simulink model "SensorFusion_Controller_Model"  (R2025a)
settings: Solver=VariableStepAuto  StartTime=0.0  StopTime=inf  FixedStep=1  RelTol=1e-3
undefined symbols (not defined in the file): DiscIntNeverNeededParam
libraries: simulink x17
(part 2 of 4)

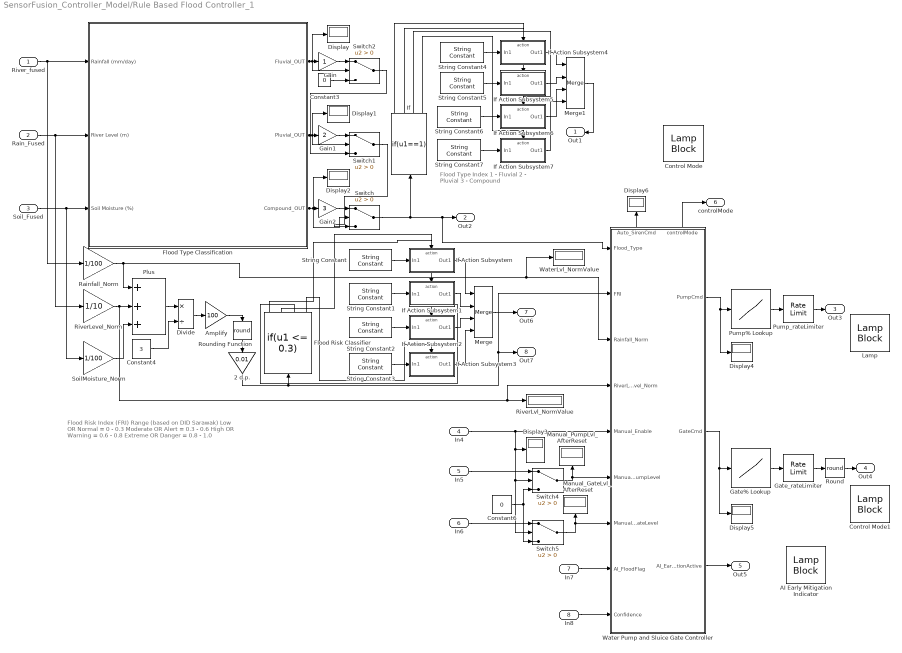
== system SensorFusion_Controller_Model/Rule Based Flood Controller_1 ==
  note: Flood Risk Index (FRI) Range (based on DID Sarawak)
      |
      | Low OR		Normal = 0 - 0.3
      | Moderate OR	Alert = 0.3 - 0.6
      | High OR		Warning = 0.6 - 0.8
      | Extreme OR 	Danger = 0.8 - 1.0
  note: Flood Type Index
      | 1 - Fluvial
      | 2 - Pluvial
      | 3 - Compound
  River_fused : Inport
  Rain_Fused : Inport  Port=2
  Soil_Fused : Inport  Port=3
  In4 : Inport  Port=4
  In5 : Inport  Port=5
  In6 : Inport  Port=6
  In7 : Inport  Port=7
  In8 : Inport  Port=8
  2 d.p. : Gain  Gain=0.01
  AI Early Mitigation Indicator : LampBlock  LabelPosition=Hide  DefaultColor=[192.0, 192.0, 192.0]
  Amplify : Gain  Gain=100
  Constant3 : Constant  Value=0
  Constant4 : Constant  Value=3
  Constant6 : Constant  Value=0
  Control Mode : LampBlock  LabelPosition=Hide  DefaultColor=[192.0, 192.0, 192.0]
  Control Mode1 : LampBlock  LabelPosition=Hide  DefaultColor=[192.0, 192.0, 192.0]
  Display{,1..6} (7 alike) : Display
  Divide : Product  Inputs=*/
  Flood Risk Classifier : If  IfExpression=u1 <= 0.3  ElseIfExpressions=u1 <= 0.6,u1 < 0.8
  Flood Type Classification : Subsystem
  Gain : Gain
  Gain1 : Gain  Gain=2
  Gain2 : Gain  Gain=3
  Gate% Lookup : Lookup_n-D  NumberOfTableDimensions=1  BreakpointsForDimension1=[0 1 2 3]  Table=[0 30 70 100]  InternalRulePriority=Speed  RndMeth=Simplest
  Gate_rateLimiter : RateLimiter  SampleTimeMode=inherited
  If : If  IfExpression=u1==1  ElseIfExpressions=u1==2,u1==3
  If Action Subsystem : Subsystem  TreatAsAtomicUnit=on
  If Action Subsystem1 : Subsystem  TreatAsAtomicUnit=on
  If Action Subsystem2 : Subsystem  TreatAsAtomicUnit=on
  If Action Subsystem3 : Subsystem  TreatAsAtomicUnit=on
  If Action Subsystem4 : Subsystem  TreatAsAtomicUnit=on
  If Action Subsystem5 : Subsystem  TreatAsAtomicUnit=on
  If Action Subsystem6 : Subsystem  TreatAsAtomicUnit=on
  If Action Subsystem7 : Subsystem  TreatAsAtomicUnit=on
  Lamp : LampBlock  LabelPosition=Hide  DefaultColor=[192.0, 192.0, 192.0]
  Manual_GateLvl_AfterReset : Display
  Manual_PumpLvl_AfterReset : Display
  Merge : Merge  Inputs=4
  Merge1 : Merge  Inputs=4
  Plus : Sum  Inputs=+++
  Pump% Lookup : Lookup_n-D  NumberOfTableDimensions=1  BreakpointsForDimension1=[0 1 2 3]  Table=[0 30 70 100]  InternalRulePriority=Speed  RndMeth=Simplest
  Pump_rateLimiter : RateLimiter  RisingSlewLimit=20  FallingSlewLimit=-30  SampleTimeMode=inherited
  Rainfall_Norm : Gain  Gain=1/100
  RiverLevel_Norm : Gain  Gain=1/10
  RiverLvl_NormValue : Display
  Round : Rounding  Operator=round
  Rounding Function : Rounding  Operator=round
  SoilMoisture_Norm : Gain  Gain=1/100
  String Constant : StringConstant  String="\"NORMAL\""
  String Constant1 : StringConstant  String="\"ALERT\""
  String Constant2 : StringConstant  String="\"WARNING\""
  String Constant3 : StringConstant  String="\"DANGER\""
  String Constant4 : StringConstant  String="\"FLUVIAL\""
  String Constant5 : StringConstant  String="\"PLUVIAL\""
  String Constant6 : StringConstant  String="\"COMPOUND\""
  String Constant7 : StringConstant  String="\"SAFE\""
  Switch{,1..2,4..5} (5 alike) : Switch  Criteria=u2 > Threshold  SaturateOnIntegerOverflow=off  InputSameDT=off
  Water Pump and Sluice Gate Controller : Stateflow chart  TreatAsAtomicUnit=on
      settings: PortSchema="{\"entries\":[{\"content\":{\"sides\":[{\"content\":{\"connectorIds\":[\"In2\",\"In1\",\"In8\",\"In9\",\"In3\",\"In5\",\"In4\",\"In6\",\"In7\"]},\"type\":\"ConnectorPlacement.EquallySpacedRectSide\",\"uuid\":\"f2c8d520-50f7-4f0f-a2cf-48793db073c2\"},{\"content\":{\"connectorIds\":[\"Out1\",\"Out2\",\"Out5\"],\"side\":\"RIGHT\"},\"type\":\"ConnectorPlacement.EquallySpacedRectSide\",\"uuid\":\"5649f6ce-feb7-45bc-b5a3-9e67182959d5\"},{\"content\":{\"connectorIds\":[\"Out3\",\"Out4\"],\"side\":\"TOP\"},\"type\":\"ConnectorPlacement.EquallySpacedRectSide\",\"uuid\":\"5d953d1b-f348-4b99-981e-4266d38d1676\"}]},\"type\":\"ConnectorPlacement.EquallySpacedConnector\",\"uuid\":\"2b0f672a-dc23-486c-8ba1-c7509a856d5e\"}],\"packageUris\":[\"http://schema.mathworks.com/mf0/Connector/R2020b\"],\"version\":\"1.0\"}"
  WaterLvl_NormValue : Display
  Out1 : Outport
  Out2 : Outport  Port=2
  Out3 : Outport  Port=3
  Out4 : Outport  Port=4
  Out5 : Outport  Port=5
  controlMode : Outport  Port=6
  Out6 : Outport  Port=7
  Out7 : Outport  Port=8
  wires:
  If/3 -> If Action Subsystem6/Action
  RiverLevel_Norm/1 -> Plus/2, RiverLvl_NormValue/1, Water Pump and Sluice Gate Controller/9(RiverLevel_Norm)
  String Constant2/1 -> If Action Subsystem2/1(In1)
  Flood Risk Classifier/2 -> If Action Subsystem1/Action
  If Action Subsystem3/1(Out1) -> Merge/4
  Soil_Fused/1 -> SoilMoisture_Norm/1, Flood Type Classification/3(Soil Moisture (%))
  Rain_Fused/1 -> RiverLevel_Norm/1, Flood Type Classification/2(River Level (m))
  String Constant1/1 -> If Action Subsystem1/1(In1)
  Flood Risk Classifier/4 -> If Action Subsystem3/Action
  If Action Subsystem7/1(Out1) -> Merge1/4
  In7/1 -> Water Pump and Sluice Gate Controller/6(AI_FloodFlag)
  Amplify/1 -> Rounding Function/1
  Constant3/1 -> Switch2/3
  Merge1/1 -> Out1/1
  Water Pump and Sluice Gate Controller/1(PumpCmd) -> Display4/1, Pump% Lookup/1
  Water Pump and Sluice Gate Controller/5(AI_EarlyMitigationActive) -> Out5/1
  Switch4/1 -> Water Pump and Sluice Gate Controller/5(Manual_PumpLevel), Manual_PumpLvl_AfterReset/1
  String Constant5/1 -> If Action Subsystem5/1(In1)
  String Constant3/1 -> If Action Subsystem3/1(In1)
  Flood Risk Classifier/1 -> If Action Subsystem/Action
  String Constant4/1 -> If Action Subsystem4/1(In1)
  Water Pump and Sluice Gate Controller/2(GateCmd) -> Display5/1, Gate% Lookup/1
  In6/1 -> Switch5/1
  If/4 -> If Action Subsystem7/Action
  String Constant6/1 -> If Action Subsystem6/1(In1)
  Divide/1 -> Amplify/1
  If Action Subsystem2/1(Out1) -> Merge/3
  Gain1/1 -> Switch1/1
  Flood Risk Classifier/3 -> If Action Subsystem2/Action
  Gain/1 -> Switch2/1
  Water Pump and Sluice Gate Controller/3(Auto_SirenCmd) -> Display6/1
  Gain2/1 -> Switch/1
  If Action Subsystem4/1(Out1) -> Merge1/1
  Switch/1 -> Out2/1, Water Pump and Sluice Gate Controller/2(Flood_Type), If/1
  Switch2/1 -> Switch1/3
  If Action Subsystem5/1(Out1) -> Merge1/2
  Flood Type Classification/3(Compound_OUT) -> Display2/1, Switch/2, Gain2/1
  If Action Subsystem6/1(Out1) -> Merge1/3
  Flood Type Classification/2(Pluvial_OUT) -> Display1/1, Switch1/2, Gain1/1
  2 d.p./1 -> Out7/1, Water Pump and Sluice Gate Controller/1(FRI), Flood Risk Classifier/1
  If Action Subsystem/1(Out1) -> Merge/1
  River_fused/1 -> Flood Type Classification/1(Rainfall (mm/day)), Rainfall_Norm/1
  Switch5/1 -> Water Pump and Sluice Gate Controller/4(Manual_GateLevel), Manual_GateLvl_AfterReset/1
  Switch1/1 -> Switch/3
  If Action Subsystem1/1(Out1) -> Merge/2
  Gate_rateLimiter/1 -> Round/1
  Merge/1 -> Out6/1
  If/1 -> If Action Subsystem4/Action
  Plus/1 -> Divide/1
  Pump% Lookup/1 -> Pump_rateLimiter/1
  Water Pump and Sluice Gate Controller/4(controlMode) -> controlMode/1
  Constant4/1 -> Divide/2
  Rainfall_Norm/1 -> Water Pump and Sluice Gate Controller/8(Rainfall_Norm), WaterLvl_NormValue/1, Plus/1
  String Constant7/1 -> If Action Subsystem7/1(In1)
  In8/1 -> Water Pump and Sluice Gate Controller/7(Confidence)
  If/2 -> If Action Subsystem5/Action
  In4/1 -> Switch5/2, Switch4/2, Display3/1, Water Pump and Sluice Gate Controller/3(Manual_Enable)
  Constant6/1 -> Switch5/3, Switch4/3
  SoilMoisture_Norm/1 -> Plus/3
  String Constant/1 -> If Action Subsystem/1(In1)
  Gate% Lookup/1 -> Gate_rateLimiter/1
  In5/1 -> Switch4/1
  Rounding Function/1 -> 2 d.p./1
  Flood Type Classification/1(Fluvial_OUT) -> Display/1, Switch2/2, Gain/1
  Pump_rateLimiter/1 -> Out3/1
  Round/1 -> Out4/1

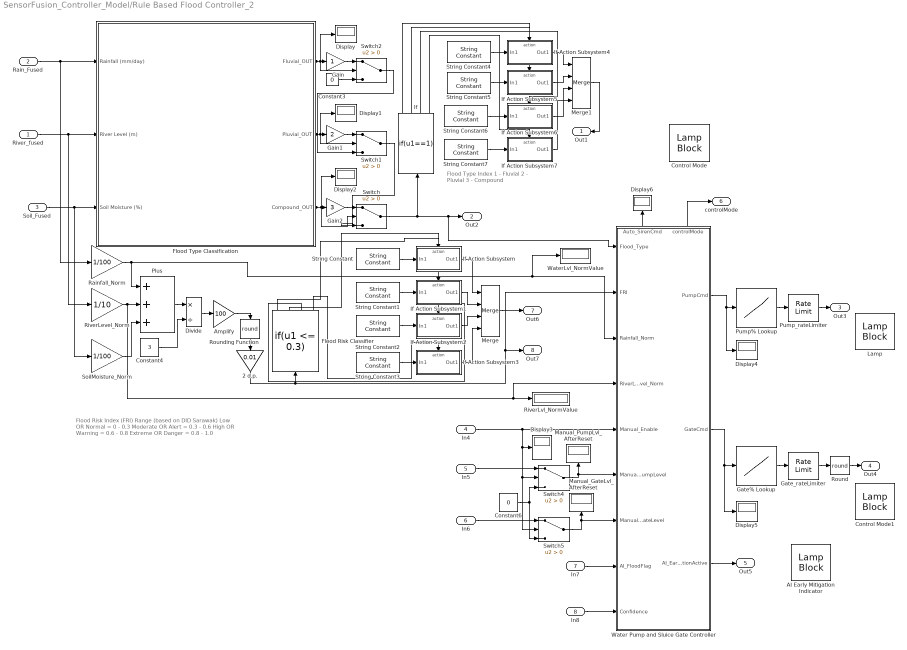
== system SensorFusion_Controller_Model/Rule Based Flood Controller_2 ==
  note: Flood Risk Index (FRI) Range (based on DID Sarawak)
      |
      | Low OR		Normal = 0 - 0.3
      | Moderate OR	Alert = 0.3 - 0.6
      | High OR		Warning = 0.6 - 0.8
      | Extreme OR 	Danger = 0.8 - 1.0
  note: Flood Type Index
      | 1 - Fluvial
      | 2 - Pluvial
      | 3 - Compound
  River_fused : Inport
  Rain_Fused : Inport  Port=2
  Soil_Fused : Inport  Port=3
  In4 : Inport  Port=4
  In5 : Inport  Port=5
  In6 : Inport  Port=6
  In7 : Inport  Port=7
  In8 : Inport  Port=8
  2 d.p. : Gain  Gain=0.01
  AI Early Mitigation Indicator : LampBlock  LabelPosition=Hide  DefaultColor=[192.0, 192.0, 192.0]
  Amplify : Gain  Gain=100
  Constant3 : Constant  Value=0
  Constant4 : Constant  Value=3
  Constant6 : Constant  Value=0
  Control Mode : LampBlock  LabelPosition=Hide  DefaultColor=[192.0, 192.0, 192.0]
  Control Mode1 : LampBlock  LabelPosition=Hide  DefaultColor=[192.0, 192.0, 192.0]
  Display{,1..6} (7 alike) : Display
  Divide : Product  Inputs=*/
  Flood Risk Classifier : If  IfExpression=u1 <= 0.3  ElseIfExpressions=u1 <= 0.6,u1 < 0.8
  Flood Type Classification : Subsystem
  Gain : Gain
  Gain1 : Gain  Gain=2
  Gain2 : Gain  Gain=3
  Gate% Lookup : Lookup_n-D  NumberOfTableDimensions=1  BreakpointsForDimension1=[0 1 2 3]  Table=[0 30 70 100]  InternalRulePriority=Speed  RndMeth=Simplest
  Gate_rateLimiter : RateLimiter  SampleTimeMode=inherited
  If : If  IfExpression=u1==1  ElseIfExpressions=u1==2,u1==3
  If Action Subsystem : Subsystem  TreatAsAtomicUnit=on
  If Action Subsystem1 : Subsystem  TreatAsAtomicUnit=on
  If Action Subsystem2 : Subsystem  TreatAsAtomicUnit=on
  If Action Subsystem3 : Subsystem  TreatAsAtomicUnit=on
  If Action Subsystem4 : Subsystem  TreatAsAtomicUnit=on
  If Action Subsystem5 : Subsystem  TreatAsAtomicUnit=on
  If Action Subsystem6 : Subsystem  TreatAsAtomicUnit=on
  If Action Subsystem7 : Subsystem  TreatAsAtomicUnit=on
  Lamp : LampBlock  LabelPosition=Hide  DefaultColor=[192.0, 192.0, 192.0]
  Manual_GateLvl_AfterReset : Display
  Manual_PumpLvl_AfterReset : Display
  Merge : Merge  Inputs=4
  Merge1 : Merge  Inputs=4
  Plus : Sum  Inputs=+++
  Pump% Lookup : Lookup_n-D  NumberOfTableDimensions=1  BreakpointsForDimension1=[0 1 2 3]  Table=[0 30 70 100]  InternalRulePriority=Speed  RndMeth=Simplest
  Pump_rateLimiter : RateLimiter  RisingSlewLimit=20  FallingSlewLimit=-30  SampleTimeMode=inherited
  Rainfall_Norm : Gain  Gain=1/100
  RiverLevel_Norm : Gain  Gain=1/10
  RiverLvl_NormValue : Display
  Round : Rounding  Operator=round
  Rounding Function : Rounding  Operator=round
  SoilMoisture_Norm : Gain  Gain=1/100
  String Constant : StringConstant  String="\"NORMAL\""
  String Constant1 : StringConstant  String="\"ALERT\""
  String Constant2 : StringConstant  String="\"WARNING\""
  String Constant3 : StringConstant  String="\"DANGER\""
  String Constant4 : StringConstant  String="\"FLUVIAL\""
  String Constant5 : StringConstant  String="\"PLUVIAL\""
  String Constant6 : StringConstant  String="\"COMPOUND\""
  String Constant7 : StringConstant  String="\"SAFE\""
  Switch{,1..2,4..5} (5 alike) : Switch  Criteria=u2 > Threshold  SaturateOnIntegerOverflow=off  InputSameDT=off
  Water Pump and Sluice Gate Controller : Stateflow chart  TreatAsAtomicUnit=on
      settings: PortSchema="{\"entries\":[{\"content\":{\"sides\":[{\"content\":{\"connectorIds\":[\"In2\",\"In1\",\"In8\",\"In9\",\"In3\",\"In5\",\"In4\",\"In6\",\"In7\"]},\"type\":\"ConnectorPlacement.EquallySpacedRectSide\",\"uuid\":\"f2c8d520-50f7-4f0f-a2cf-48793db073c2\"},{\"content\":{\"connectorIds\":[\"Out1\",\"Out2\",\"Out5\"],\"side\":\"RIGHT\"},\"type\":\"ConnectorPlacement.EquallySpacedRectSide\",\"uuid\":\"5649f6ce-feb7-45bc-b5a3-9e67182959d5\"},{\"content\":{\"connectorIds\":[\"Out3\",\"Out4\"],\"side\":\"TOP\"},\"type\":\"ConnectorPlacement.EquallySpacedRectSide\",\"uuid\":\"5d953d1b-f348-4b99-981e-4266d38d1676\"}]},\"type\":\"ConnectorPlacement.EquallySpacedConnector\",\"uuid\":\"2b0f672a-dc23-486c-8ba1-c7509a856d5e\"}],\"packageUris\":[\"http://schema.mathworks.com/mf0/Connector/R2020b\"],\"version\":\"1.0\"}"
  WaterLvl_NormValue : Display
  Out1 : Outport
  Out2 : Outport  Port=2
  Out3 : Outport  Port=3
  Out4 : Outport  Port=4
  Out5 : Outport  Port=5
  controlMode : Outport  Port=6
  Out6 : Outport  Port=7
  Out7 : Outport  Port=8
  wires:
  If/3 -> If Action Subsystem6/Action
  RiverLevel_Norm/1 -> Plus/2, RiverLvl_NormValue/1, Water Pump and Sluice Gate Controller/9(RiverLevel_Norm)
  String Constant2/1 -> If Action Subsystem2/1(In1)
  Flood Risk Classifier/2 -> If Action Subsystem1/Action
  If Action Subsystem3/1(Out1) -> Merge/4
  Soil_Fused/1 -> SoilMoisture_Norm/1, Flood Type Classification/3(Soil Moisture (%))
  River_fused/1 -> Flood Type Classification/2(River Level (m)), RiverLevel_Norm/1
  String Constant1/1 -> If Action Subsystem1/1(In1)
  Flood Risk Classifier/4 -> If Action Subsystem3/Action
  If Action Subsystem7/1(Out1) -> Merge1/4
  In7/1 -> Water Pump and Sluice Gate Controller/6(AI_FloodFlag)
  Amplify/1 -> Rounding Function/1
  Constant3/1 -> Switch2/3
  Merge1/1 -> Out1/1
  Water Pump and Sluice Gate Controller/1(PumpCmd) -> Display4/1, Pump% Lookup/1
  Water Pump and Sluice Gate Controller/5(AI_EarlyMitigationActive) -> Out5/1
  Switch4/1 -> Water Pump and Sluice Gate Controller/5(Manual_PumpLevel), Manual_PumpLvl_AfterReset/1
  String Constant5/1 -> If Action Subsystem5/1(In1)
  String Constant3/1 -> If Action Subsystem3/1(In1)
  Flood Risk Classifier/1 -> If Action Subsystem/Action
  String Constant4/1 -> If Action Subsystem4/1(In1)
  Water Pump and Sluice Gate Controller/2(GateCmd) -> Display5/1, Gate% Lookup/1
  In6/1 -> Switch5/1
  If/4 -> If Action Subsystem7/Action
  String Constant6/1 -> If Action Subsystem6/1(In1)
  Divide/1 -> Amplify/1
  If Action Subsystem2/1(Out1) -> Merge/3
  Gain1/1 -> Switch1/1
  Flood Risk Classifier/3 -> If Action Subsystem2/Action
  Gain/1 -> Switch2/1
  Water Pump and Sluice Gate Controller/3(Auto_SirenCmd) -> Display6/1
  Gain2/1 -> Switch/1
  If Action Subsystem4/1(Out1) -> Merge1/1
  Switch/1 -> Out2/1, Water Pump and Sluice Gate Controller/2(Flood_Type), If/1
  Switch2/1 -> Switch1/3
  If Action Subsystem5/1(Out1) -> Merge1/2
  Flood Type Classification/3(Compound_OUT) -> Display2/1, Switch/2, Gain2/1
  If Action Subsystem6/1(Out1) -> Merge1/3
  Flood Type Classification/2(Pluvial_OUT) -> Display1/1, Switch1/2, Gain1/1
  2 d.p./1 -> Out7/1, Water Pump and Sluice Gate Controller/1(FRI), Flood Risk Classifier/1
  If Action Subsystem/1(Out1) -> Merge/1
  Rain_Fused/1 -> Rainfall_Norm/1, Flood Type Classification/1(Rainfall (mm/day))
  Switch5/1 -> Water Pump and Sluice Gate Controller/4(Manual_GateLevel), Manual_GateLvl_AfterReset/1
  Switch1/1 -> Switch/3
  If Action Subsystem1/1(Out1) -> Merge/2
  Gate_rateLimiter/1 -> Round/1
  Merge/1 -> Out6/1
  If/1 -> If Action Subsystem4/Action
  Plus/1 -> Divide/1
  Pump% Lookup/1 -> Pump_rateLimiter/1
  Water Pump and Sluice Gate Controller/4(controlMode) -> controlMode/1
  Constant4/1 -> Divide/2
  Rainfall_Norm/1 -> Water Pump and Sluice Gate Controller/8(Rainfall_Norm), WaterLvl_NormValue/1, Plus/1
  String Constant7/1 -> If Action Subsystem7/1(In1)
  In8/1 -> Water Pump and Sluice Gate Controller/7(Confidence)
  If/2 -> If Action Subsystem5/Action
  In4/1 -> Switch5/2, Switch4/2, Display3/1, Water Pump and Sluice Gate Controller/3(Manual_Enable)
  Constant6/1 -> Switch5/3, Switch4/3
  SoilMoisture_Norm/1 -> Plus/3
  String Constant/1 -> If Action Subsystem/1(In1)
  Gate% Lookup/1 -> Gate_rateLimiter/1
  In5/1 -> Switch4/1
  Rounding Function/1 -> 2 d.p./1
  Flood Type Classification/1(Fluvial_OUT) -> Display/1, Switch2/2, Gain/1
  Pump_rateLimiter/1 -> Out3/1
  Round/1 -> Out4/1

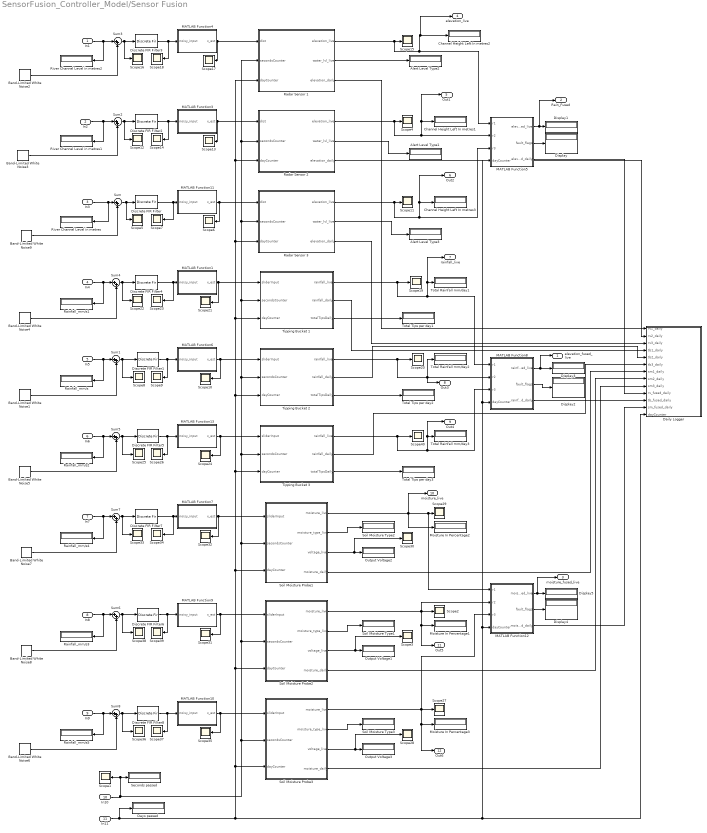
== system SensorFusion_Controller_Model/Sensor Fusion ==
  In1 : Inport
  In2 : Inport  Port=2
  In3 : Inport  Port=3
  In4 : Inport  Port=4
  In5 : Inport  Port=5
  In6 : Inport  Port=6
  In7 : Inport  Port=7
  In8 : Inport  Port=8
  In9 : Inport  Port=9
  In10 : Inport  Port=10
  In11 : Inport  Port=11
  Alert Level Type1 : Display
  Alert Level Type2 : Display
  Alert Level Type3 : Display
  Band-Limited White Noise{1,4..8} (6 alike) : simulink/Sources/Band-Limited White Noise  Cov=1e-10  Ts=1  seed=[12345]
  Band-Limited White Noise2 : simulink/Sources/Band-Limited White Noise  Cov=1e-4  Ts=1  seed=[12345]
  Band-Limited White Noise3 : simulink/Sources/Band-Limited White Noise  Cov=1e-4  Ts=1  seed=[12345]
  Band-Limited White Noise9 : simulink/Sources/Band-Limited White Noise  Cov=1e-4  Ts=1  seed=[12345]
  Channel Height Left In metres1 : Display
  Channel Height Left In metres2 : Display
  Channel Height Left In metres3 : Display
  Daily Logger : MATLAB Function  TreatAsAtomicUnit=on
  Days passed : Display
  Discrete FIR Filter : DiscreteFir  Coefficients=[0.1 0.1 0.1 0.1 0.1 0.1 0.1 0.1 0.1 0.1]
  Discrete FIR Filter{1,4..8} (6 alike) : DiscreteFir
  Discrete FIR Filter2 : DiscreteFir  Coefficients=[0.1 0.1 0.1 0.1 0.1 0.1 0.1 0.1 0.1 0.1]
  Discrete FIR Filter3 : DiscreteFir  Coefficients=[0.1 0.1 0.1 0.1 0.1 0.1 0.1 0.1 0.1 0.1]
  Display{,1..5} (6 alike) : Display
  MATLAB Function1 : MATLAB Function  TreatAsAtomicUnit=on
  MATLAB Function10 : MATLAB Function  TreatAsAtomicUnit=on
  MATLAB Function11 : MATLAB Function  TreatAsAtomicUnit=on
  MATLAB Function12 : MATLAB Function  TreatAsAtomicUnit=on
  MATLAB Function13 : MATLAB Function  TreatAsAtomicUnit=on
  MATLAB Function3 : MATLAB Function  TreatAsAtomicUnit=on
  MATLAB Function4 : MATLAB Function  TreatAsAtomicUnit=on
  MATLAB Function5 : MATLAB Function  TreatAsAtomicUnit=on
  MATLAB Function6 : MATLAB Function  TreatAsAtomicUnit=on
  MATLAB Function7 : MATLAB Function  TreatAsAtomicUnit=on
  MATLAB Function8 : MATLAB Function  TreatAsAtomicUnit=on
  MATLAB Function9 : MATLAB Function  TreatAsAtomicUnit=on
  Moisture In Percentage1 : Display
  Moisture In Percentage2 : Display
  Moisture In Percentage3 : Display
  Output Voltage1 : Display
  Output Voltage2 : Display
  Output Voltage3 : Display
  Radar Sensor 1 : MATLAB Function  TreatAsAtomicUnit=on
  Radar Sensor 2 : MATLAB Function  TreatAsAtomicUnit=on
  Radar Sensor 3 : MATLAB Function  TreatAsAtomicUnit=on
  Rainfall_mm/s{,1..5} (6 alike) : Display
  River Channel Level in metres : Display
  River Channel Level in metres1 : Display
  River Channel Level in metres2 : Display
  Scope{1..40} (40 alike) : Scope
      Scope1 settings: ActiveDisplayYMinimum=-10799.875  ActiveDisplayYMaximum=97198.875
      Scope10 settings: ActiveDisplayYMinimum=-0.04719  ActiveDisplayYMaximum=0.05304  DataLoggingVariableName=ScopeData22
      Scope11 settings: ActiveDisplayYMinimum=1.11854  ActiveDisplayYMaximum=5.0416  DataLoggingVariableName=ScopeData23
      Scope12 settings: ActiveDisplayYMinimum=3.01528  ActiveDisplayYMaximum=3.9355  DataLoggingVariableName=ScopeData24
      Scope13 settings: ActiveDisplayYMinimum=-0.048  ActiveDisplayYMaximum=4.10573  DataLoggingVariableName=ScopeData25
      Scope14 settings: ActiveDisplayYMinimum=-0.04802  ActiveDisplayYMaximum=4.10586  DataLoggingVariableName=ScopeData26
      Scope15 settings: ActiveDisplayYMinimum=0.62281  ActiveDisplayYMaximum=4.37524  DataLoggingVariableName=ScopeData27
      Scope16 settings: ActiveDisplayYMinimum=3.99995  ActiveDisplayYMaximum=4.00005  DataLoggingVariableName=ScopeData9
      Scope17 settings: ActiveDisplayYMinimum=-0.04993  ActiveDisplayYMaximum=4.45793  DataLoggingVariableName=ScopeData10
      Scope18 settings: ActiveDisplayYMinimum=-0.05025  ActiveDisplayYMaximum=4.4608  DataLoggingVariableName=ScopeData28
      Scope19 settings: ActiveDisplayYMinimum=-8.4  ActiveDisplayYMaximum=75.6  DataLoggingVariableName=ScopeData29
      Scope2 settings: ActiveDisplayYMinimum=-11.5  ActiveDisplayYMaximum=103.5  DataLoggingVariableName=ScopeData30
      Scope20 settings: ActiveDisplayYMinimum=-1.825  ActiveDisplayYMaximum=16.425  DataLoggingVariableName=ScopeData31
      Scope21 settings: ActiveDisplayYMinimum=-0.00015  ActiveDisplayYMaximum=0.00137  DataLoggingVariableName=ScopeData32
      Scope22 settings: ActiveDisplayYMinimum=-0.13163  ActiveDisplayYMaximum=0.12145  DataLoggingVariableName=ScopeData33
      Scope23 settings: ActiveDisplayYMinimum=-0.00019  ActiveDisplayYMaximum=0.00139  DataLoggingVariableName=ScopeData5
      Scope24 settings: ActiveDisplayYMinimum=-0.04719  ActiveDisplayYMaximum=0.05304  DataLoggingVariableName=ScopeData34
      Scope25 settings: ActiveDisplayYMinimum=-0.13163  ActiveDisplayYMaximum=0.12145  DataLoggingVariableName=ScopeData35
      Scope26 settings: ActiveDisplayYMinimum=-0.08478  ActiveDisplayYMaximum=0.09119  DataLoggingVariableName=ScopeData36
      Scope27 settings: ActiveDisplayYMinimum=-1  ActiveDisplayYMaximum=1  DataLoggingVariableName=ScopeData7
      Scope28 settings: ActiveDisplayYMinimum=0.47959  ActiveDisplayYMaximum=0.68376  DataLoggingVariableName=ScopeData8
      Scope29 settings: ActiveDisplayYMinimum=-14.25  ActiveDisplayYMaximum=128.25  DataLoggingVariableName=ScopeData11
      Scope3 settings: ActiveDisplayYMinimum=0.47959  ActiveDisplayYMaximum=0.68376  DataLoggingVariableName=ScopeData6
      Scope30 settings: ActiveDisplayYMinimum=0.43225  ActiveDisplayYMaximum=1.10997  DataLoggingVariableName=ScopeData12
      Scope31 settings: ActiveDisplayYMinimum=-0.00015  ActiveDisplayYMaximum=0.00137  DataLoggingVariableName=ScopeData13
      Scope32 settings: ActiveDisplayYMinimum=-0.04719  ActiveDisplayYMaximum=0.05304  DataLoggingVariableName=ScopeData14
      Scope33 settings: ActiveDisplayYMinimum=-0.13163  ActiveDisplayYMaximum=0.12145  DataLoggingVariableName=ScopeData15
      Scope34 settings: ActiveDisplayYMinimum=-0.08478  ActiveDisplayYMaximum=0.09119  DataLoggingVariableName=ScopeData16
      Scope35 settings: ActiveDisplayYMinimum=0  ActiveDisplayYMaximum=0.00135  DataLoggingVariableName=ScopeData17
      Scope36 settings: ActiveDisplayYMinimum=-0.13163  ActiveDisplayYMaximum=0.12145  DataLoggingVariableName=ScopeData18
      Scope37 settings: ActiveDisplayYMinimum=-0.08478  ActiveDisplayYMaximum=0.09119  DataLoggingVariableName=ScopeData19
      Scope38 settings: ActiveDisplayYMinimum=-0.13163  ActiveDisplayYMaximum=0.12145  DataLoggingVariableName=ScopeData20
      Scope39 settings: ActiveDisplayYMinimum=-0.08478  ActiveDisplayYMaximum=0.09119  DataLoggingVariableName=ScopeData21
      Scope4 settings: ActiveDisplayYMinimum=1.11854  ActiveDisplayYMaximum=5.0416  DataLoggingVariableName=ScopeData37
      Scope40 settings: ActiveDisplayYMinimum=-9.85  ActiveDisplayYMaximum=88.65  DataLoggingVariableName=ScopeData4
      Scope5 settings: ActiveDisplayYMinimum=3.01528  ActiveDisplayYMaximum=3.9355  DataLoggingVariableName=ScopeData38
      Scope6 settings: ActiveDisplayYMinimum=-0.05012  ActiveDisplayYMaximum=4.45962  DataLoggingVariableName=ScopeData39
      Scope7 settings: ActiveDisplayYMinimum=-0.03899  ActiveDisplayYMaximum=3.30223  DataLoggingVariableName=ScopeData3
      Scope8 settings: ActiveDisplayYMinimum=-0.13163  ActiveDisplayYMaximum=0.12145
      Scope9 settings: ActiveDisplayYMinimum=-0.08478  ActiveDisplayYMaximum=0.09119  DataLoggingVariableName=ScopeData2
  Seconds passed : Display
  Soil Moisture Probe1 : MATLAB Function  TreatAsAtomicUnit=on
  Soil Moisture Probe2 : MATLAB Function  TreatAsAtomicUnit=on
  Soil Moisture Probe3 : MATLAB Function  TreatAsAtomicUnit=on
  Soil Moisture Type1 : Display
  Soil Moisture Type2 : Display
  Soil Moisture Type3 : Display
  Sum{,1..8} (9 alike) : Sum  Inputs=|++
  Tipping Bucket 1 : MATLAB Function  TreatAsAtomicUnit=on
  Tipping Bucket 2 : MATLAB Function  TreatAsAtomicUnit=on
  Tipping Bucket 3 : MATLAB Function  TreatAsAtomicUnit=on
  Total Rainfall mm/day1 : Display
  Total Rainfall mm/day2 : Display
  Total Rainfall mm/day3 : Display
  Total Tips per day1 : Display
  Total Tips per day2 : Display
  Total Tips per day3 : Display
  elevation_fused_live : Outport
  Rain_Fused : Outport  Port=2
  moisture_fused_live : Outport  Port=3
  elevation_live : Outport  Port=4
  Out1 : Outport  Port=5
  Out2 : Outport  Port=6
  rainfall_live : Outport  Port=7
  Out3 : Outport  Port=8
  Out4 : Outport  Port=9
  moisture_live : Outport  Port=10
  Out5 : Outport  Port=11
  Out6 : Outport  Port=12
  wires:
  MATLAB Function6/1(x_est) -> Tipping Bucket 2/1(sliderInput), Scope10/1
  Band-Limited White Noise9/1 -> Sum/2
  MATLAB Function8/3(rainfall_fused_daily) -> Daily Logger/11(tb_fused_daily)
  MATLAB Function5/3(elevation_fused_daily) -> Daily Logger/10(rv_fused_daily)
  Discrete FIR Filter5/1 -> MATLAB Function13/1(noisy_input), Scope26/1
  In6/1 -> Sum5/1, Rainfall_mm/s2/1
  Tipping Bucket 2/3(totalTipsDaily) -> Total Tips per day2/1
  Discrete FIR Filter/1 -> Scope7/1, MATLAB Function11/1(noisy_input)
  In10/1 -> Seconds passed/1, Scope1/1, Soil Moisture Probe3/2(secondsCounter), Soil Moisture Probe2/2(secondsCounter), Tipping Bucket 3/2(secondsCounter), Tipping Bucket 2/2(secondsCounter), Tipping Bucket 1/2(secondsCounter), Radar Sensor 3/2(secondsCounter), Radar Sensor 2/2(secondsCounter), Radar Sensor 1/2(secondsCounter), Soil Moisture Probe1/2(secondsCounter)
  MATLAB Function12/2(fault_flags) -> Display4/1
  In5/1 -> Sum1/1, Rainfall_mm/s/1
  Sum2/1 -> Discrete FIR Filter2/1, Scope12/1
  Radar Sensor 2/3(elevation_daily) -> Daily Logger/2(rv2_daily)
  Soil Moisture Probe2/2(moisture_type_live) -> Soil Moisture Type1/1
  Discrete FIR Filter2/1 -> MATLAB Function3/1(noisy_input), Scope14/1
  Band-Limited White Noise4/1 -> Sum4/2
  MATLAB Function1/1(x_est) -> Tipping Bucket 1/1(sliderInput), Scope21/1
  In2/1 -> Sum2/1, River Channel Level in metres1/1
  Tipping Bucket 1/2(rainfall_daily) -> Daily Logger/4(tb1_daily)
  Soil Moisture Probe1/1(moisture_live) -> Moisture In Percentage2/1, moisture_live/1, MATLAB Function12/1(r1), Scope29/1
  MATLAB Function5/2(fault_flags) -> Display/1
  MATLAB Function8/1(rainfall_fused_live) -> elevation_fused_live/1, Display3/1
  MATLAB Function10/1(x_est) -> Soil Moisture Probe3/1(sliderInput), Scope35/1
  Tipping Bucket 2/2(rainfall_daily) -> Daily Logger/5(tb2_daily)
  Discrete FIR Filter1/1 -> MATLAB Function6/1(noisy_input), Scope9/1
  In3/1 -> Sum/1, River Channel Level in metres/1
  Radar Sensor 1/1(elevation_live) -> Scope15/1, elevation_live/1, Channel Height Left In metres2/1, MATLAB Function5/1(r1)
  Band-Limited White Noise3/1 -> Sum2/2
  In8/1 -> Sum6/1, Rainfall_mm/s3/1
  Band-Limited White Noise1/1 -> Sum1/2
  Tipping Bucket 1/3(totalTipsDaily) -> Total Tips per day1/1
  MATLAB Function4/1(x_est) -> Radar Sensor 1/1(dist), Scope17/1
  Tipping Bucket 3/3(totalTipsDaily) -> Total Tips per day3/1
  MATLAB Function9/1(x_est) -> Soil Moisture Probe2/1(sliderInput), Scope31/1
  In1/1 -> Sum3/1, River Channel Level in metres2/1
  Band-Limited White Noise5/1 -> Sum5/2
  Band-Limited White Noise2/1 -> Sum3/2
  Soil Moisture Probe3/3(voltage_live) -> Scope28/1, Output Voltage3/1
  Radar Sensor 3/1(elevation_live) -> Scope11/1, MATLAB Function5/3(r3), Out2/1, Channel Height Left In metres3/1
  Sum/1 -> Discrete FIR Filter/1, Scope5/1
  Sum6/1 -> Scope38/1, Discrete FIR Filter6/1
  Tipping Bucket 3/1(rainfall_live) -> MATLAB Function8/3(r3), Out4/1, Total Rainfall mm/day3/1, Scope40/1
  Soil Moisture Probe3/4(moisture_daily) -> Daily Logger/9(sm3_daily)
  Radar Sensor 3/2(water_lvl_live) -> Alert Level Type3/1
  Tipping Bucket 2/1(rainfall_live) -> Out3/1, Total Rainfall mm/day2/1, MATLAB Function8/2(r2), Scope20/1
  Soil Moisture Probe2/4(moisture_daily) -> Daily Logger/8(sm2_daily)
  Discrete FIR Filter6/1 -> MATLAB Function9/1(noisy_input), Scope39/1
  Band-Limited White Noise6/1 -> Sum8/2
  MATLAB Function12/1(moisture_fused_live) -> moisture_fused_live/1, Display5/1
  Soil Moisture Probe2/3(voltage_live) -> Scope3/1, Output Voltage1/1
  Sum7/1 -> Scope33/1, Discrete FIR Filter7/1
  Discrete FIR Filter7/1 -> MATLAB Function7/1(noisy_input), Scope34/1
  Radar Sensor 2/1(elevation_live) -> Scope4/1, Out1/1, Channel Height Left In metres1/1, MATLAB Function5/2(r2)
  Sum4/1 -> Scope22/1, Discrete FIR Filter4/1
  Sum3/1 -> Discrete FIR Filter3/1, Scope16/1
  Radar Sensor 3/3(elevation_daily) -> Daily Logger/3(rv3_daily)
  MATLAB Function5/1(elevation_fused_live) -> Rain_Fused/1, Display1/1
  In11/1 -> MATLAB Function12/4(dayCounter), MATLAB Function5/4(dayCounter), MATLAB Function8/4(dayCounter), Daily Logger/13(dayCounter), Soil Moisture Probe3/3(dayCounter), Soil Moisture Probe2/3(dayCounter), Tipping Bucket 3/3(dayCounter), Tipping Bucket 2/3(dayCounter), Tipping Bucket 1/3(dayCounter), Radar Sensor 3/3(dayCounter), Radar Sensor 2/3(dayCounter), Radar Sensor 1/3(dayCounter), Soil Moisture Probe1/3(dayCounter), Days passed/1
  MATLAB Function13/1(x_est) -> Tipping Bucket 3/1(sliderInput), Scope24/1
  In7/1 -> Sum7/1, Rainfall_mm/s4/1
  Sum1/1 -> Scope8/1, Discrete FIR Filter1/1
  Soil Moisture Probe1/4(moisture_daily) -> Daily Logger/7(sm1_daily)
  Radar Sensor 1/2(water_lvl_live) -> Alert Level Type2/1
  Radar Sensor 2/2(water_lvl_live) -> Alert Level Type1/1
  Discrete FIR Filter8/1 -> MATLAB Function10/1(noisy_input), Scope37/1
  MATLAB Function12/3(moisture_fused_daily) -> Daily Logger/12(sm_fused_daily)
  Tipping Bucket 3/2(rainfall_daily) -> Daily Logger/6(tb3_daily)
  Soil Moisture Probe3/2(moisture_type_live) -> Soil Moisture Type3/1
  Radar Sensor 1/3(elevation_daily) -> Daily Logger/1(rv1_daily)
  Band-Limited White Noise8/1 -> Sum6/2
  MATLAB Function11/1(x_est) -> Radar Sensor 3/1(dist), Scope6/1
  MATLAB Function8/2(fault_flags) -> Display2/1
  Soil Moisture Probe1/2(moisture_type_live) -> Soil Moisture Type2/1
  Sum8/1 -> Scope36/1, Discrete FIR Filter8/1
  Sum5/1 -> Scope25/1, Discrete FIR Filter5/1
  In4/1 -> Sum4/1, Rainfall_mm/s1/1
  MATLAB Function3/1(x_est) -> Radar Sensor 2/1(dist), Scope13/1
  Soil Moisture Probe1/3(voltage_live) -> Output Voltage2/1, Scope30/1
  Soil Moisture Probe3/1(moisture_live) -> MATLAB Function12/3(r3), Scope27/1, Out6/1, Moisture In Percentage3/1
  Band-Limited White Noise7/1 -> Sum7/2
  Discrete FIR Filter3/1 -> Scope18/1, MATLAB Function4/1(noisy_input)
  Soil Moisture Probe2/1(moisture_live) -> MATLAB Function12/2(r2), Out5/1, Moisture In Percentage1/1, Scope2/1
  MATLAB Function7/1(x_est) -> Scope32/1, Soil Moisture Probe1/1(sliderInput)
  Discrete FIR Filter4/1 -> MATLAB Function1/1(noisy_input), Scope23/1
  In9/1 -> Sum8/1, Rainfall_mm/s5/1
  Tipping Bucket 1/1(rainfall_live) -> rainfall_live/1, Total Rainfall mm/day1/1, MATLAB Function8/1(r1), Scope19/1

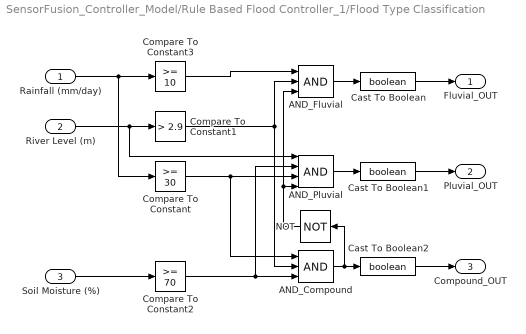
== system SensorFusion_Controller_Model/Rule Based Flood Controller_1/Flood Type Classification ==
  Rainfall (mm/day) : Inport
  River Level (m) : Inport  Port=2
  Soil Moisture (%) : Inport  Port=3
  AND_Compound : Logic  Inputs=3  IconShape=distinctive  AllPortsSameDT=off  OutDataTypeStr=boolean
  AND_Fluvial : Logic  Inputs=3  IconShape=distinctive  AllPortsSameDT=off  OutDataTypeStr=boolean
  AND_Pluvial : Logic  Inputs=4  IconShape=distinctive  AllPortsSameDT=off  OutDataTypeStr=boolean
  Cast To Boolean : DataTypeConversion  OutDataTypeStr=boolean  SaturateOnIntegerOverflow=off  RndMeth=Floor
  Cast To Boolean1 : DataTypeConversion  OutDataTypeStr=boolean  SaturateOnIntegerOverflow=off  RndMeth=Floor
  Cast To Boolean2 : DataTypeConversion  OutDataTypeStr=boolean  SaturateOnIntegerOverflow=off  RndMeth=Floor
  Compare To Constant : simulink/Logic and Bit Operations/Compare To Constant  relop=>=  const=30  OutDataTypeStr=boolean
  Compare To Constant1 : simulink/Logic and Bit Operations/Compare To Constant  relop=>  const=2.9  OutDataTypeStr=boolean
  Compare To Constant2 : simulink/Logic and Bit Operations/Compare To Constant  relop=>=  const=70  OutDataTypeStr=boolean
  Compare To Constant3 : simulink/Logic and Bit Operations/Compare To Constant  relop=>=  const=10  OutDataTypeStr=boolean
  NOT : Logic  Operator=NOT  IconShape=distinctive  AllPortsSameDT=off  OutDataTypeStr=boolean
  Fluvial_OUT : Outport
  Pluvial_OUT : Outport  Port=2
  Compound_OUT : Outport  Port=3
  wires:
  Rainfall (mm/day)/1 -> Compare To Constant/1, Compare To Constant3/1
  River Level (m)/1 -> AND_Pluvial/1, Compare To Constant1/1
  Soil Moisture (%)/1 -> Compare To Constant2/1
  Compare To Constant/1 -> AND_Compound/1, AND_Pluvial/3
  Compare To Constant1/1 -> AND_Fluvial/2, AND_Compound/2
  Compare To Constant2/1 -> AND_Pluvial/2, AND_Compound/3
  Compare To Constant3/1 -> AND_Fluvial/1
  AND_Fluvial/1 -> Cast To Boolean/1
  Cast To Boolean/1 -> Fluvial_OUT/1
  Cast To Boolean1/1 -> Pluvial_OUT/1
  AND_Compound/1 -> NOT/1, Cast To Boolean2/1
  AND_Pluvial/1 -> Cast To Boolean1/1
  Cast To Boolean2/1 -> Compound_OUT/1
  NOT/1 -> AND_Fluvial/3, AND_Pluvial/4

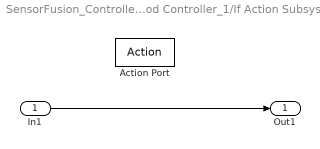
== system SensorFusion_Controller_Model/Rule Based Flood Controller_1/If Action Subsystem ==
  In1 : Inport
  Action Port : ActionPort  ActionPortLabel=if(u1 <= 0.3)
  Out1 : Outport
  wires:
  In1/1 -> Out1/1

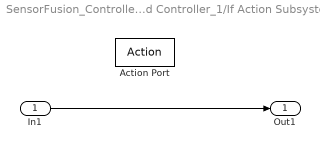
== system SensorFusion_Controller_Model/Rule Based Flood Controller_1/If Action Subsystem1 ==
  In1 : Inport
  Action Port : ActionPort  ActionPortLabel=elseif(u1 <= 0.6)
  Out1 : Outport
  wires:
  In1/1 -> Out1/1

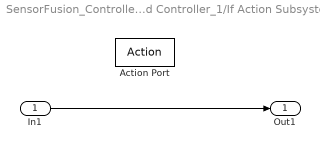
== system SensorFusion_Controller_Model/Rule Based Flood Controller_1/If Action Subsystem2 ==
  In1 : Inport
  Action Port : ActionPort  ActionPortLabel=elseif(u1 < 0.8)
  Out1 : Outport
  wires:
  In1/1 -> Out1/1

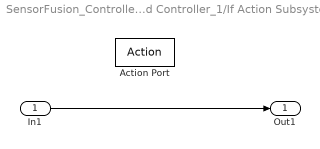
== system SensorFusion_Controller_Model/Rule Based Flood Controller_1/If Action Subsystem3 ==
  In1 : Inport
  Action Port : ActionPort  ActionPortLabel=else
  Out1 : Outport
  wires:
  In1/1 -> Out1/1

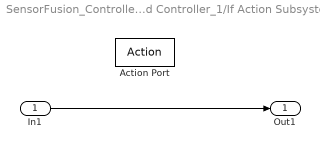
== system SensorFusion_Controller_Model/Rule Based Flood Controller_1/If Action Subsystem4 ==
  In1 : Inport
  Action Port : ActionPort  ActionPortLabel=if(u1==1)
  Out1 : Outport
  wires:
  In1/1 -> Out1/1

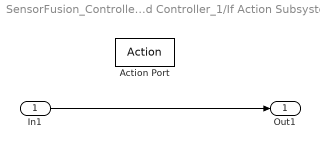
== system SensorFusion_Controller_Model/Rule Based Flood Controller_1/If Action Subsystem5 ==
  In1 : Inport
  Action Port : ActionPort  ActionPortLabel=elseif(u1==2)
  Out1 : Outport
  wires:
  In1/1 -> Out1/1

== system SensorFusion_Controller_Model/Rule Based Flood Controller_1/If Action Subsystem6 ==
  In1 : Inport
  Action Port : ActionPort  ActionPortLabel=elseif(u1==3)
  Out1 : Outport
  wires:
  In1/1 -> Out1/1

== system SensorFusion_Controller_Model/Rule Based Flood Controller_1/If Action Subsystem7 ==
  In1 : Inport
  Action Port : ActionPort  ActionPortLabel=else
  Out1 : Outport
  wires:
  In1/1 -> Out1/1

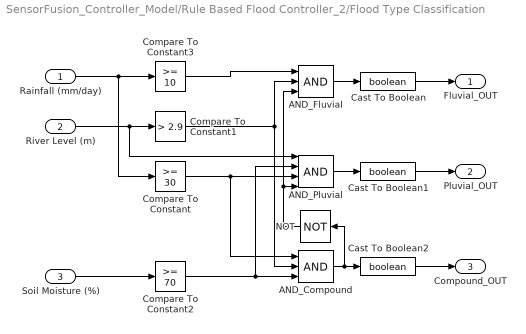
== system SensorFusion_Controller_Model/Rule Based Flood Controller_2/Flood Type Classification ==
  Rainfall (mm/day) : Inport
  River Level (m) : Inport  Port=2
  Soil Moisture (%) : Inport  Port=3
  AND_Compound : Logic  Inputs=3  IconShape=distinctive  AllPortsSameDT=off  OutDataTypeStr=boolean
  AND_Fluvial : Logic  Inputs=3  IconShape=distinctive  AllPortsSameDT=off  OutDataTypeStr=boolean
  AND_Pluvial : Logic  Inputs=4  IconShape=distinctive  AllPortsSameDT=off  OutDataTypeStr=boolean
  Cast To Boolean : DataTypeConversion  OutDataTypeStr=boolean  SaturateOnIntegerOverflow=off  RndMeth=Floor
  Cast To Boolean1 : DataTypeConversion  OutDataTypeStr=boolean  SaturateOnIntegerOverflow=off  RndMeth=Floor
  Cast To Boolean2 : DataTypeConversion  OutDataTypeStr=boolean  SaturateOnIntegerOverflow=off  RndMeth=Floor
  Compare To Constant : simulink/Logic and Bit Operations/Compare To Constant  relop=>=  const=30  OutDataTypeStr=boolean
  Compare To Constant1 : simulink/Logic and Bit Operations/Compare To Constant  relop=>  const=2.9  OutDataTypeStr=boolean
  Compare To Constant2 : simulink/Logic and Bit Operations/Compare To Constant  relop=>=  const=70  OutDataTypeStr=boolean
  Compare To Constant3 : simulink/Logic and Bit Operations/Compare To Constant  relop=>=  const=10  OutDataTypeStr=boolean
  NOT : Logic  Operator=NOT  IconShape=distinctive  AllPortsSameDT=off  OutDataTypeStr=boolean
  Fluvial_OUT : Outport
  Pluvial_OUT : Outport  Port=2
  Compound_OUT : Outport  Port=3
  wires:
  Rainfall (mm/day)/1 -> Compare To Constant/1, Compare To Constant3/1
  River Level (m)/1 -> AND_Pluvial/1, Compare To Constant1/1
  Soil Moisture (%)/1 -> Compare To Constant2/1
  Compare To Constant/1 -> AND_Compound/1, AND_Pluvial/3
  Compare To Constant1/1 -> AND_Fluvial/2, AND_Compound/2
  Compare To Constant2/1 -> AND_Pluvial/2, AND_Compound/3
  Compare To Constant3/1 -> AND_Fluvial/1
  AND_Fluvial/1 -> Cast To Boolean/1
  Cast To Boolean/1 -> Fluvial_OUT/1
  Cast To Boolean1/1 -> Pluvial_OUT/1
  AND_Compound/1 -> NOT/1, Cast To Boolean2/1
  AND_Pluvial/1 -> Cast To Boolean1/1
  Cast To Boolean2/1 -> Compound_OUT/1
  NOT/1 -> AND_Fluvial/3, AND_Pluvial/4

== system SensorFusion_Controller_Model/Rule Based Flood Controller_2/If Action Subsystem ==
  In1 : Inport
  Action Port : ActionPort  ActionPortLabel=if(u1 <= 0.3)
  Out1 : Outport
  wires:
  In1/1 -> Out1/1

== system SensorFusion_Controller_Model/Rule Based Flood Controller_2/If Action Subsystem1 ==
  In1 : Inport
  Action Port : ActionPort  ActionPortLabel=elseif(u1 <= 0.6)
  Out1 : Outport
  wires:
  In1/1 -> Out1/1

== system SensorFusion_Controller_Model/Rule Based Flood Controller_2/If Action Subsystem2 ==
  In1 : Inport
  Action Port : ActionPort  ActionPortLabel=elseif(u1 < 0.8)
  Out1 : Outport
  wires:
  In1/1 -> Out1/1

== system SensorFusion_Controller_Model/Rule Based Flood Controller_2/If Action Subsystem3 ==
  In1 : Inport
  Action Port : ActionPort  ActionPortLabel=else
  Out1 : Outport
  wires:
  In1/1 -> Out1/1

== system SensorFusion_Controller_Model/Rule Based Flood Controller_2/If Action Subsystem4 ==
  In1 : Inport
  Action Port : ActionPort  ActionPortLabel=if(u1==1)
  Out1 : Outport
  wires:
  In1/1 -> Out1/1

== system SensorFusion_Controller_Model/Rule Based Flood Controller_2/If Action Subsystem5 ==
  In1 : Inport
  Action Port : ActionPort  ActionPortLabel=elseif(u1==2)
  Out1 : Outport
  wires:
  In1/1 -> Out1/1

== system SensorFusion_Controller_Model/Rule Based Flood Controller_2/If Action Subsystem6 ==
  In1 : Inport
  Action Port : ActionPort  ActionPortLabel=elseif(u1==3)
  Out1 : Outport
  wires:
  In1/1 -> Out1/1

== system SensorFusion_Controller_Model/Rule Based Flood Controller_2/If Action Subsystem7 ==
  In1 : Inport
  Action Port : ActionPort  ActionPortLabel=else
  Out1 : Outport
  wires:
  In1/1 -> Out1/1

== matlab function SensorFusion_Controller_Model/MATLAB Function2 ==
  data: secondsCounter output; dayCounter output; u input
function [secondsCounter, dayCounter] = timerFcn(u)

persistent seconds day
if isempty(seconds)
    seconds = 0;
end

if isempty(day)
    day = 0;
end

% count seconds to full day
seconds = seconds + 1;

% full day passed (24 hours = 86400 sec)
if mod(seconds,86400 ) == 0
    day = day + 1;
end

% output
secondsCounter = mod(seconds,86400);
dayCounter = day;

== matlab function SensorFusion_Controller_Model/Sensor Fusion/Radar Sensor 2 ==
  data: dist input; elevation_live output; secondsCounter input; dayCounter input; water_lvl_live output; elevation_daily output
function [elevation_live, water_lvl_live, elevation_daily] = riverElevationSensor(dist, secondsCounter, dayCounter)

% INPUTS:
% dist - radar-measured distance from sensor to water surface (m) comes from the dashboard slider input
% secondsCounter - current second within the day (0 to 86399), from timer
% dayCounter- how many full days have passed, from timer
%
% OUTPUTS (LIVE that updates every timestep, use these for dashboard):
% elevation_live - current smoothed river water elevation in metres
% water_lvl_live - current water level status string (live, for dashboard)
%
% OUTPUTS (DAILY AVERAGE - updates once per day rollover, use for logger):
% elevation_daily - average river elevation across the entire previous day (m) computed as running sum 
% over 86400 seconds
%
% HOW IT WORKS:
% the sensor converts radar distance to river elevation using a fixed reference elevation (ref_elev).
% a smoothing factor gradually moves the elevation toward the target rather than jumping instantly,
% simulating real sensor lag. Every 86400 seconds (1 day), the current live values are saved as
% the daily snapshot before the timer resets.

ref_elev = 5.0; % height of sensor mount above riverbed (metres)
% water elevation = ref_elev - dist
MIN_ELEV = 0.0; % river physically cannot be below 0m
MAX_ELEV = 4.0; % maximum valid river level as defined by project spec

persistent prevSec prevDay elevation elevation_daily_store daily_sum daily_count

% initialise persistent variables
if isempty(prevSec), prevSec = 0; end
if isempty(prevDay), prevDay = 0; end
if isempty(elevation), elevation = ref_elev - dist; end
if isempty(elevation_daily_store), elevation_daily_store = 0; end
if isempty(daily_sum), daily_sum = 0; end
if isempty(daily_count), daily_count = 0; end

% time delta calculation
deltaT = secondsCounter - prevSec;
if deltaT <= 0
    deltaT = 1; % guard against zero or negative delta on reset tick
end

% target_elev is where the reading should be based on current dist input
target_elev = ref_elev - dist;

% clamp the target to valid physical range to prevents the slider going out of range
target_elev = max(MIN_ELEV, min(MAX_ELEV, target_elev));

% gradually move elevation toward target (smoothing factor = 100)
% a higher denominator = slower/smoother response to input changes
rate = (target_elev - elevation) / 100;
elevation = elevation + rate * deltaT;
elevation = max(MIN_ELEV, min(MAX_ELEV, elevation));

% Water level classification (based on live elevation) Thresholds (metres):
% elevation > 2.05 = Normal
% 1.70 < elevation <= 2.05 = Alert
% elevation <= 1.70 = Critical
if elevation > 2.05
    water_lvl_str = "Normal";
elseif elevation > 1.70
    water_lvl_str = "Alert";
else
    water_lvl_str = "Critical";
end

% add current elevation to running sum for daily average calculation
% Simulink calls this function every timestep so daily_sum accumulates all readings across the day,
% daily_count tracks how many readings taken
daily_sum   = daily_sum + elevation;
daily_count = daily_count + 1;

% daily average when the day counter increments
% when dayCounter changes, it means 86400s have passed and the timer reset for new day
if double(dayCounter) ~= double(prevDay)
    if daily_count > 0
        elevation_daily_store = daily_sum / daily_count; % true daily average
    end
    daily_sum   = 0; % reset accumulator for new day
    daily_count = 0; % reset sample counter for new day
    prevDay = double(dayCounter);
end

% update state for next timestep
prevSec = secondsCounter;

% assign outputs
% live outputs to the dashboard signals
elevation_live = elevation;
water_lvl_live = water_lvl_str;

% daily average output to the dailyLogger block
elevation_daily = elevation_daily_store;

end

== matlab function SensorFusion_Controller_Model/Sensor Fusion/Radar Sensor 3 ==
  data: dist input; elevation_live output; secondsCounter input; dayCounter input; water_lvl_live output; elevation_daily output
function [elevation_live, water_lvl_live, elevation_daily] = riverElevationSensor(dist, secondsCounter, dayCounter)

% INPUTS:
% dist - radar-measured distance from sensor to water surface (m) comes from the dashboard slider input
% secondsCounter - current second within the day (0 to 86399), from timer
% dayCounter- how many full days have passed, from timer
%
% OUTPUTS (LIVE that updates every timestep, use these for dashboard):
% elevation_live - current smoothed river water elevation in metres
% water_lvl_live - current water level status string (live, for dashboard)
%
% OUTPUTS (DAILY AVERAGE - updates once per day rollover, use for logger):
% elevation_daily - average river elevation across the entire previous day (m) computed as running sum 
% over 86400 seconds
%
% HOW IT WORKS:
% the sensor converts radar distance to river elevation using a fixed reference elevation (ref_elev).
% a smoothing factor gradually moves the elevation toward the target rather than jumping instantly,
% simulating real sensor lag. Every 86400 seconds (1 day), the current live values are saved as
% the daily snapshot before the timer resets.

ref_elev = 5.0; % height of sensor mount above riverbed (metres)
% water elevation = ref_elev - dist
MIN_ELEV = 0.0; % river physically cannot be below 0m
MAX_ELEV = 4.0; % maximum valid river level as defined by project spec

persistent prevSec prevDay elevation elevation_daily_store daily_sum daily_count

% initialise persistent variables
if isempty(prevSec), prevSec = 0; end
if isempty(prevDay), prevDay = 0; end
if isempty(elevation), elevation = ref_elev - dist; end
if isempty(elevation_daily_store), elevation_daily_store = 0; end
if isempty(daily_sum), daily_sum = 0; end
if isempty(daily_count), daily_count = 0; end

% time delta calculation
deltaT = secondsCounter - prevSec;
if deltaT <= 0
    deltaT = 1; % guard against zero or negative delta on reset tick
end

% target_elev is where the reading should be based on current dist input
target_elev = ref_elev - dist;

% clamp the target to valid physical range to prevents the slider going out of range
target_elev = max(MIN_ELEV, min(MAX_ELEV, target_elev));

% gradually move elevation toward target (smoothing factor = 100)
% a higher denominator = slower/smoother response to input changes
rate = (target_elev - elevation) / 100;
elevation = elevation + rate * deltaT;
elevation = max(MIN_ELEV, min(MAX_ELEV, elevation));

% Water level classification (based on live elevation) Thresholds (metres):
% elevation > 2.05 = Normal
% 1.70 < elevation <= 2.05 = Alert
% elevation <= 1.70 = Critical
if elevation > 2.05
    water_lvl_str = "Normal";
elseif elevation > 1.70
    water_lvl_str = "Alert";
else
    water_lvl_str = "Critical";
end

% add current elevation to running sum for daily average calculation
% Simulink calls this function every timestep so daily_sum accumulates all readings across the day,
% daily_count tracks how many readings taken
daily_sum   = daily_sum + elevation;
daily_count = daily_count + 1;

% daily average when the day counter increments
% when dayCounter changes, it means 86400s have passed and the timer reset for new day
if double(dayCounter) ~= double(prevDay)
    if daily_count > 0
        elevation_daily_store = daily_sum / daily_count; % true daily average
    end
    daily_sum   = 0; % reset accumulator for new day
    daily_count = 0; % reset sample counter for new day
    prevDay = double(dayCounter);
end

% update state for next timestep
prevSec = secondsCounter;

% assign outputs
% live outputs to the dashboard signals
elevation_live = elevation;
water_lvl_live = water_lvl_str;

% daily average output to the dailyLogger block
elevation_daily = elevation_daily_store;

end

== matlab function SensorFusion_Controller_Model/Sensor Fusion/MATLAB Function4 ==
  data: noisy_input input; x_est output
function x_est = kalmanFilter(noisy_input)

persistent x P
if isempty(x), x = noisy_input; end
if isempty(P), P = 1; end


Q = 1e-4;   % process noise covariance
R = 1e-3;   % measurement noise covariance
% R > Q : filter trusts its own prediction slightly more than noise
% measurement

% prediction
x_pred = x;
P_pred = P + Q;

% update
K = P_pred / (P_pred + R);
x = x_pred + K*(noisy_input - x_pred);
P = (1 - K)*P_pred;

x_est = max(0, x);
